simulink model "Exercise5_marc"  (R2018b)
settings: Solver=VariableStepAuto  StartTime=0.0  StopTime=1  RelTol=1e-3
libraries: arduinolib x2
settings Model: Creator=tuxtorn  LastModifiedBy=tuxtorn

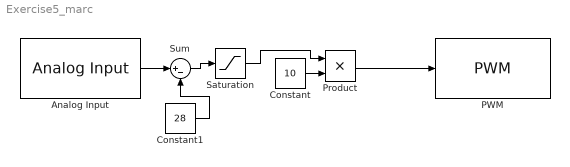
== system Exercise5_marc ==
  Analog Input : arduinolib/Analog Input  pinNumber=4  ReadResultsOnly=off  ConversionTriggerSource=Software  ExternalTriggerType=uint32(0)  OutputDataType=uint16  EnableConversionCompleteNotify=off  EnableOuputStatus=off  SampleTime=1  blockPlatform=arduino
  Constant : Constant  Value=10
  Constant1 : Constant  Value=28
  PWM : arduinolib/PWM  pinNumber=8  EnableInputFrequency=off  InitialFrequency=2000  InitialDutyCycle=0  NotificationType=None  blockPlatform=arduino
  Product : Product
  Saturation : Saturate  UpperLimit=Inf  LowerLimit=0
  Sum : Sum  Inputs=|+-
  wires:
  Product/1 -> PWM/1
  Constant/1 -> Product/2
  Constant1/1 -> Sum/2
  Analog Input/1 -> Sum/1
  Sum/1 -> Saturation/1
  Saturation/1 -> Product/1
